simulink model "ALL_toghether"  (R2020b)
settings: Solver=ode1  StartTime=0.0  StopTime=50  FixedStep=0.001  RelTol=1e-3
values from neighbouring files (symbols this model uses):
  A = [0 -pi/16 0;pi/16 0 3*pi/16;0 0 0]    [feedbackControllerFinal.m]
  A_original1 = 1.2*A    [feedbackControllerFinal.m]
  A_original2 = 5*A    [feedbackControllerFinal.m]
  B = [1/2 1/2;0 0;1/0.15 -1/0.15]    [feedbackControllerFinal.m]
  C = [1 0 0;0 1 0]    [feedbackControllerFinal.m]
  F = -40    [feedbackControllerFinal.m]
  G_closeLoop = inv(C*inv(-(A-B*K1))*B)    [feedbackControllerFinal.m]
  K1 = place(A, B, [-30 -1+4.899*i -1-4.899*i])    [feedbackControllerFinal.m]
  K_f = K_bar(:,1:3)    [feedbackControllerFinal.m]
  Ka = K_bar(:,4:5)    [feedbackControllerFinal.m]
  L = L'    [feedbackControllerFinal.m]
  L_R = [1 -400]    [feedbackControllerFinal.m]
  Q1 = [1 0; 0 1; -0.5031 67.9061]    [feedbackControllerFinal.m]
  Q2 = [0 0 6.7909]'    [feedbackControllerFinal.m]
  T = lyap(-F, A, -L_R*C)    [feedbackControllerFinal.m]
settings Model: Creator=maral  LastModifiedBy=BALUCH
settings DebuggingCC: ArithmeticOperatorsInVariantConditions=warning
settings SFSimCC: CustomCodeUndefinedFunction=UseInterfaceOnly

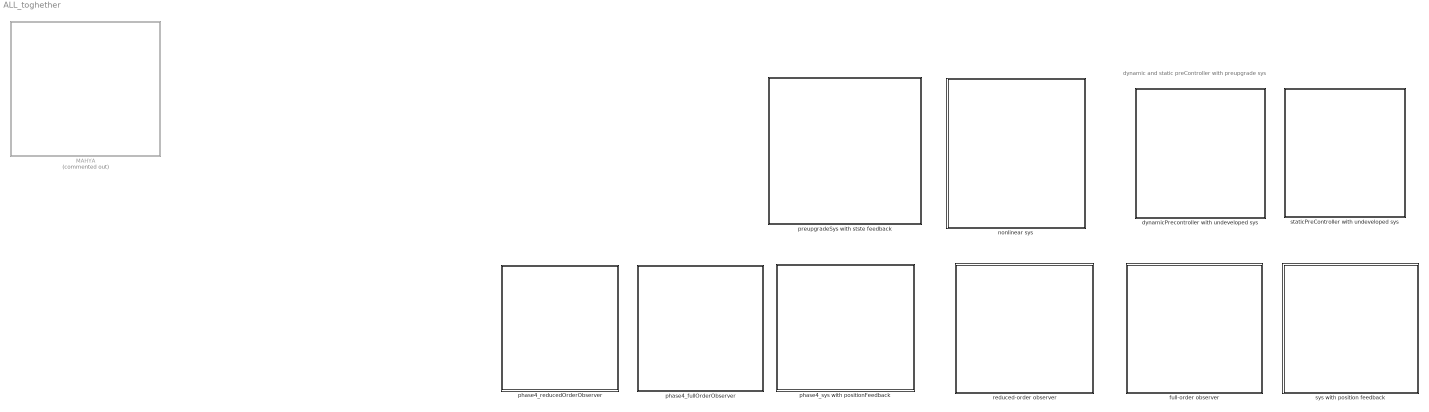
== system ALL_toghether ==
  note: dynamic and static preController with preupgrade sys
  "MAHYA " : Subsystem  Commented=on
  "dynamicPrecontroller with undeveloped sys " : Subsystem
  "full-order observer " : Subsystem
  "nonlinear sys " : Subsystem
  "phase4_fullOrderObserver " : Subsystem
  "phase4_reducedOrderObserver " : Subsystem
  "phase4_sys with positionFeedback " : Subsystem
  "preupgradeSys with stste feedback " : Subsystem
  reduced-order observer : Subsystem
  staticPreController with undeveloped sys : Subsystem
  sys with position feedback : Subsystem

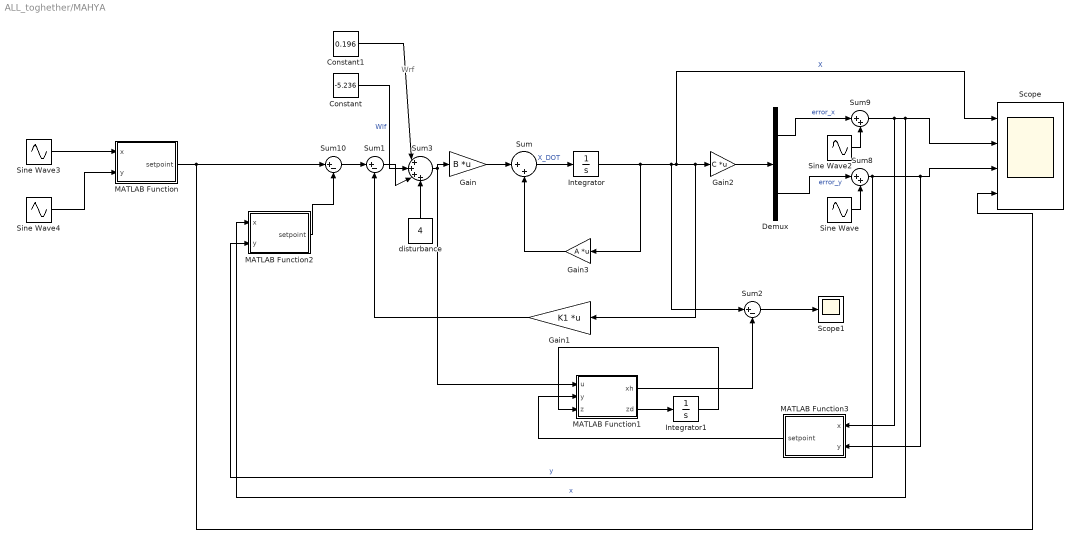
== system ALL_toghether/MAHYA  ==
  note: Wrf
  Constant : Constant  Value=-5.236
  Constant1 : Constant  Value=0.196
  Demux : Demux  Outputs=2
  Gain : Gain  Gain=B  Multiplication=Matrix(K*u)
  Gain1 : Gain  Gain=K1  Multiplication=Matrix(K*u)
  Gain2 : Gain  Gain=C  Multiplication=Matrix(K*u)
  Gain3 : Gain  Gain=A  Multiplication=Matrix(K*u)
  Integrator : Integrator
  Integrator1 : Integrator  InitialCondition=[0 0 0]
  MATLAB Function : MATLAB Function  TreatAsAtomicUnit=on
  MATLAB Function1 : MATLAB Function  TreatAsAtomicUnit=on
  MATLAB Function2 : MATLAB Function  TreatAsAtomicUnit=on
  MATLAB Function3 : MATLAB Function  TreatAsAtomicUnit=on
  Scope : Scope  NumInputPorts=4
  Scope1 : Scope
  Sine Wave : Sin  Amplitude=-3  Frequency=1/32  SampleTime=0
  Sine Wave2 : Sin  Amplitude=3  Frequency=1/32  Phase=pi/2  SampleTime=0
  Sine Wave3 : Sin  Amplitude=3  Frequency=1/30  Phase=pi/2  SampleTime=0
  Sine Wave4 : Sin  Amplitude=-3  Frequency=1/32  SampleTime=0
  Sum : Sum  Inputs=|++
  Sum1 : Sum  Inputs=|+-
  Sum10 : Sum  Inputs=|+-
  Sum2 : Sum  Inputs=|+-
  Sum3 : Sum  Inputs=|++++
  Sum8 : Sum  Inputs=|++
  Sum9 : Sum  Inputs=|++
  "disturbance " : Constant  Value=4
  wires:
  Demux/1 -> Sum9/1  "error_x"
  Sum9/1 -> MATLAB Function3/1(x), MATLAB Function2/1(x), Scope/2  "x"
  Gain3/1 -> Sum/2
  Sum8/1 -> MATLAB Function2/2(y), MATLAB Function3/2(y), Scope/3  "y"
  Gain2/1 -> Demux/1
  Sum10/1 -> Sum1/1
  MATLAB Function/1(setpoint) -> Scope/4, Sum10/1
  Integrator/1 -> Gain3/1, Sum2/1, Scope/1, Gain1/1, Gain2/1  "X"
  Gain/1 -> Sum/1
  Gain1/1 -> Sum1/2
  "disturbance "/1 -> Sum3/4
  Sum3/1 -> Gain/1, MATLAB Function1/1(u)
  Sine Wave/1 -> Sum8/2
  Sum/1 -> Integrator/1  "X_DOT"
  Sum1/1 -> Sum3/3
  Constant/1 -> Sum3/2  "Wlf"
  Sine Wave4/1 -> MATLAB Function/2(y)
  Sine Wave3/1 -> MATLAB Function/1(x)
  Sine Wave2/1 -> Sum9/2
  Constant1/1 -> Sum3/1
  MATLAB Function2/1(setpoint) -> Sum10/2
  Demux/2 -> Sum8/1  "error_y"
  MATLAB Function1/2(zd) -> Integrator1/1
  Integrator1/1 -> MATLAB Function1/3(z)
  MATLAB Function3/1(setpoint) -> MATLAB Function1/2(y)
  MATLAB Function1/1(xh) -> Sum2/2
  Sum2/1 -> Scope1/1

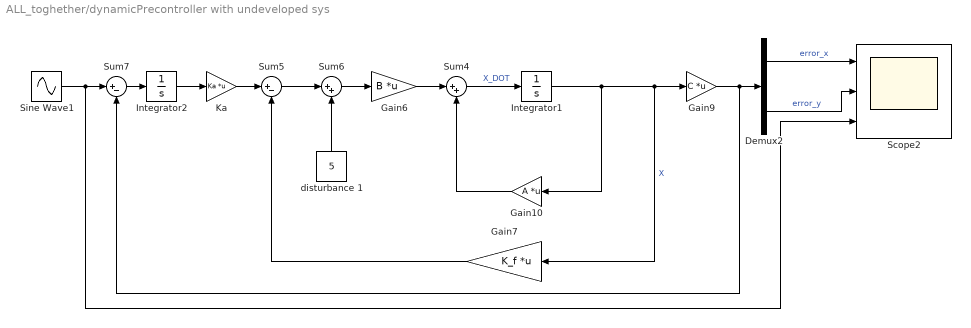
== system ALL_toghether/dynamicPrecontroller with undeveloped sys  ==
  Demux2 : Demux  Outputs=2
  Gain10 : Gain  Gain=A  Multiplication=Matrix(K*u)
  Gain6 : Gain  Gain=B  Multiplication=Matrix(K*u)
  Gain7 : Gain  Gain=K_f  Multiplication=Matrix(K*u)
  Gain9 : Gain  Gain=C  Multiplication=Matrix(K*u)
  Integrator1 : Integrator
  Integrator2 : Integrator
  "Ka " : Gain  Gain=Ka  Multiplication=Matrix(K*u)
  Scope2 : Scope  NumInputPorts=3
  Sine Wave1 : Sin  Amplitude=[1 1]  Bias=[0 0]  Frequency=[1 1]  SampleTime=0
  Sum4 : Sum  Inputs=|++
  Sum5 : Sum  Inputs=|+-
  Sum6 : Sum  Inputs=|++
  Sum7 : Sum  Inputs=|+-
  disturbance 1 : Constant  Value=5
  wires:
  Sum5/1 -> Sum6/1
  Integrator2/1 -> "Ka "/1
  Sum7/1 -> Integrator2/1
  disturbance 1/1 -> Sum6/2
  Integrator1/1 -> Gain10/1, Gain7/1, Gain9/1  "X"
  Gain7/1 -> Sum5/2
  Gain6/1 -> Sum4/1
  Gain10/1 -> Sum4/2
  Sine Wave1/1 -> Scope2/3, Sum7/1
  Demux2/2 -> Scope2/2  "error_y"
  "Ka "/1 -> Sum5/1
  Sum6/1 -> Gain6/1
  Demux2/1 -> Scope2/1  "error_x"
  Gain9/1 -> Sum7/2, Demux2/1
  Sum4/1 -> Integrator1/1  "X_DOT"

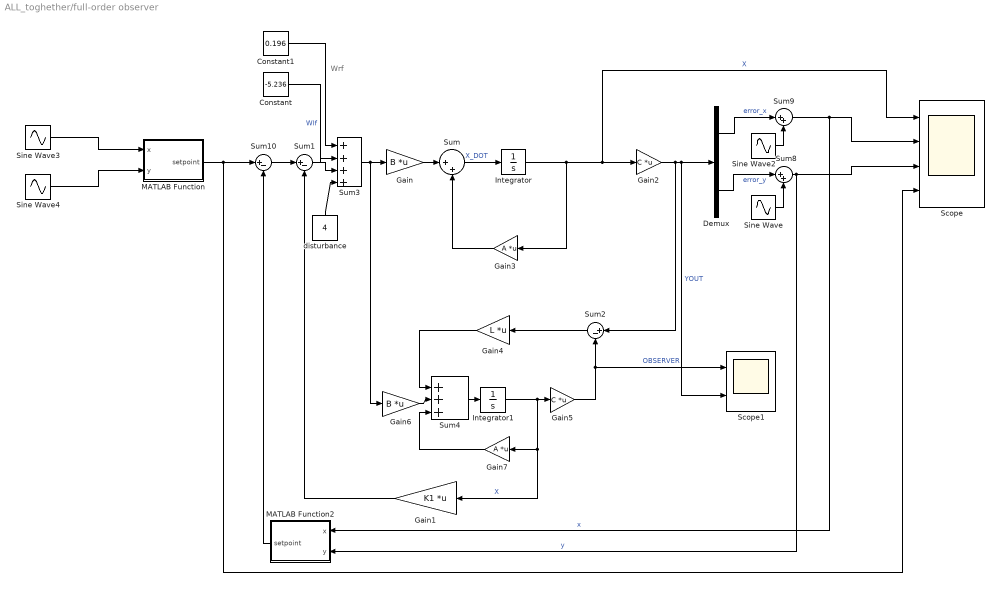
== system ALL_toghether/full-order observer  ==
  note: Wrf
  Constant : Constant  Value=-5.236
  Constant1 : Constant  Value=0.196
  Demux : Demux  Outputs=2
  Gain : Gain  Gain=B  Multiplication=Matrix(K*u)
  Gain1 : Gain  Gain=K1  Multiplication=Matrix(K*u)
  Gain2 : Gain  Gain=C  Multiplication=Matrix(K*u)
  Gain3 : Gain  Gain=A  Multiplication=Matrix(K*u)
  Gain4 : Gain  Gain=L  Multiplication=Matrix(K*u)
  Gain5 : Gain  Gain=C  Multiplication=Matrix(K*u)
  Gain6 : Gain  Gain=B  Multiplication=Matrix(K*u)
  Gain7 : Gain  Gain=A  Multiplication=Matrix(K*u)
  Integrator : Integrator  InitialCondition=[0.1 0.1 0]'
  Integrator1 : Integrator  InitialCondition=[0.4 0.4 0.5]'
  MATLAB Function : MATLAB Function  TreatAsAtomicUnit=on
  MATLAB Function2 : MATLAB Function  TreatAsAtomicUnit=on
  Scope : Scope  NumInputPorts=4
  Scope1 : Scope  NumInputPorts=2
  Sine Wave : Sin  Amplitude=-3  Frequency=pi/16  SampleTime=0
  Sine Wave2 : Sin  Amplitude=3  Frequency=pi/16  Phase=pi/2  SampleTime=0
  Sine Wave3 : Sin  Amplitude=3  Frequency=pi/16  Phase=pi/2  SampleTime=0
  Sine Wave4 : Sin  Amplitude=-3  Frequency=pi/16  SampleTime=0
  Sum : Sum  Inputs=|++
  Sum1 : Sum  Inputs=|+-
  Sum10 : Sum  Inputs=|+-
  Sum2 : Sum  Inputs=|+-
  Sum3 : Sum  Inputs=|++++
  Sum4 : Sum  Inputs=|+++
  Sum8 : Sum  Inputs=|++
  Sum9 : Sum  Inputs=|++
  "disturbance " : Constant  Value=4
  wires:
  Sum8/1 -> MATLAB Function2/2(y), Scope/3  "y"
  Constant/1 -> Sum3/2  "Wlf"
  Sum10/1 -> Sum1/1
  Sine Wave/1 -> Sum8/2
  Integrator/1 -> Gain3/1, Scope/1, Gain2/1  "X"
  Gain1/1 -> Sum1/2
  Demux/1 -> Sum9/1  "error_x"
  "disturbance "/1 -> Sum3/4
  Sum9/1 -> MATLAB Function2/1(x), Scope/2  "x"
  MATLAB Function/1(setpoint) -> Scope/4, Sum10/1
  Constant1/1 -> Sum3/1
  Sine Wave2/1 -> Sum9/2
  Sum3/1 -> Gain6/1, Gain/1
  Gain3/1 -> Sum/2
  Gain2/1 -> Sum2/1, Scope1/2, Demux/1  "YOUT"
  Sum1/1 -> Sum3/3
  Sine Wave3/1 -> MATLAB Function/1(x)
  Gain/1 -> Sum/1
  MATLAB Function2/1(setpoint) -> Sum10/2
  Demux/2 -> Sum8/1  "error_y"
  Sine Wave4/1 -> MATLAB Function/2(y)
  Sum/1 -> Integrator/1  "X_DOT"
  Gain5/1 -> Sum2/2, Scope1/1  "OBSERVER"
  Integrator1/1 -> Gain7/1, Gain1/1, Gain5/1  "X"
  Sum4/1 -> Integrator1/1
  Gain6/1 -> Sum4/2
  Gain4/1 -> Sum4/1
  Gain7/1 -> Sum4/3
  Sum2/1 -> Gain4/1

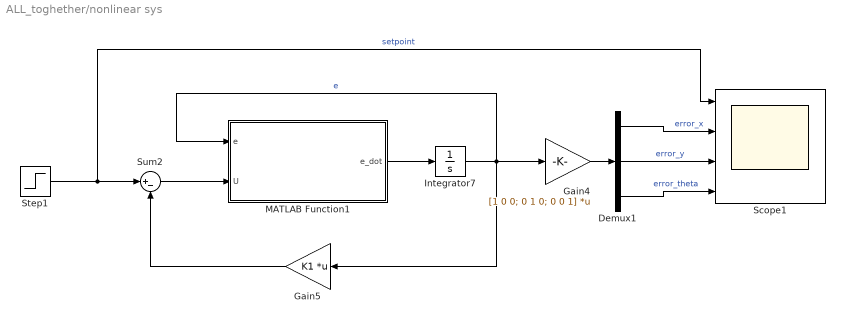
== system ALL_toghether/nonlinear sys  ==
  Demux1 : Demux  Outputs=3
  Gain4 : Gain  Gain=[1 0 0; 0 1 0; 0 0 1]  Multiplication=Matrix(K*u)
  Gain5 : Gain  Gain=K1  Multiplication=Matrix(K*u)
  Integrator7 : Integrator  InitialCondition=[0.45; -0.3; -0.3]
  MATLAB Function1 : MATLAB Function  TreatAsAtomicUnit=on
  Scope1 : Scope  NumInputPorts=4
  Step1 : Step  Time=[0;0]  Before=[0;0]  After=[0.1;0.2]  SampleTime=0
  Sum2 : Sum  Inputs=|+-
  wires:
  Sum2/1 -> MATLAB Function1/2(U)
  Gain5/1 -> Sum2/2
  Integrator7/1 -> MATLAB Function1/1(e), Gain4/1, Gain5/1  "e"
  MATLAB Function1/1(e_dot) -> Integrator7/1
  Gain4/1 -> Demux1/1
  Demux1/1 -> Scope1/2  "error_x"
  Step1/1 -> Sum2/1, Scope1/1  "setpoint"
  Demux1/2 -> Scope1/3  "error_y"
  Demux1/3 -> Scope1/4  "error_theta"

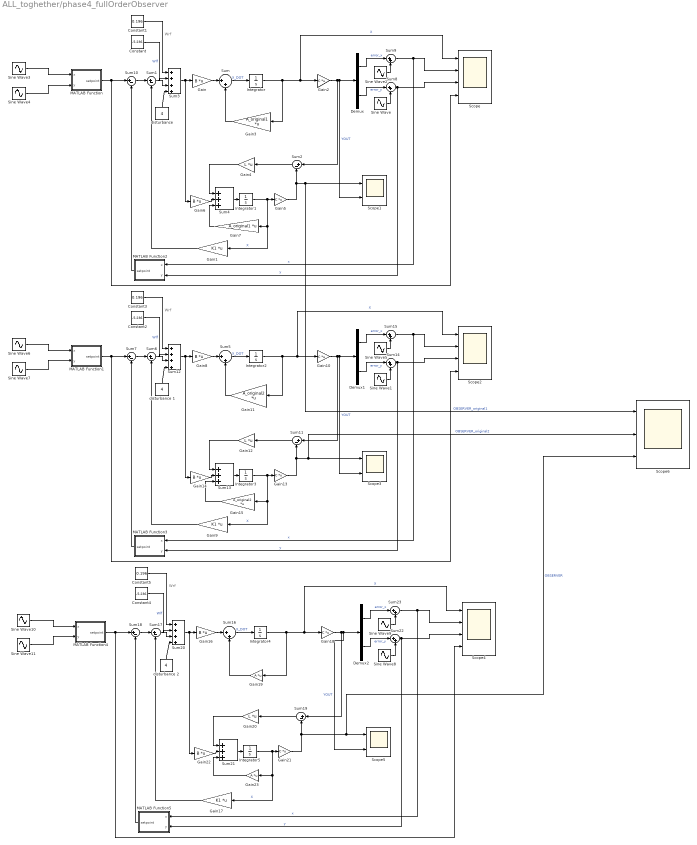
== system ALL_toghether/phase4_fullOrderObserver  ==
  note: Wrf
  note: Wrf
  note: Wrf
  Constant : Constant  Value=-5.236
  Constant1 : Constant  Value=0.196
  Constant2 : Constant  Value=-5.236
  Constant3 : Constant  Value=0.196
  Constant4 : Constant  Value=-5.236
  Constant5 : Constant  Value=0.196
  Demux : Demux  Outputs=2
  Demux1 : Demux  Outputs=2
  Demux2 : Demux  Outputs=2
  Gain{,6,8,14,16,22} (6 alike) : Gain  Gain=B  Multiplication=Matrix(K*u)
  Gain1 : Gain  Gain=K1  Multiplication=Matrix(K*u)
  Gain{2,5,10,13,18,21} (6 alike) : Gain  Gain=C  Multiplication=Matrix(K*u)
  Gain11 : Gain  Gain=A_original2  Multiplication=Matrix(K*u)
  Gain12 : Gain  Gain=L  Multiplication=Matrix(K*u)
  Gain15 : Gain  Gain=A_original2  Multiplication=Matrix(K*u)
  Gain17 : Gain  Gain=K1  Multiplication=Matrix(K*u)
  Gain19 : Gain  Gain=A  Multiplication=Matrix(K*u)
  Gain20 : Gain  Gain=L  Multiplication=Matrix(K*u)
  Gain23 : Gain  Gain=A  Multiplication=Matrix(K*u)
  Gain3 : Gain  Gain=A_original1  Multiplication=Matrix(K*u)
  Gain4 : Gain  Gain=L  Multiplication=Matrix(K*u)
  Gain7 : Gain  Gain=A_original1  Multiplication=Matrix(K*u)
  Gain9 : Gain  Gain=K1  Multiplication=Matrix(K*u)
  Integrator : Integrator  InitialCondition=[0.1 0.1 0]'
  Integrator1 : Integrator  InitialCondition=[0.4 0.4 0.5]'
  Integrator2 : Integrator  InitialCondition=[0.1 0.1 0]'
  Integrator3 : Integrator  InitialCondition=[0.4 0.4 0.5]'
  Integrator4 : Integrator  InitialCondition=[0.1 0.1 0]'
  Integrator5 : Integrator  InitialCondition=[0.4 0.4 0.5]'
  MATLAB Function : MATLAB Function  TreatAsAtomicUnit=on
  MATLAB Function1 : MATLAB Function  TreatAsAtomicUnit=on
  MATLAB Function2 : MATLAB Function  TreatAsAtomicUnit=on
  MATLAB Function3 : MATLAB Function  TreatAsAtomicUnit=on
  MATLAB Function4 : MATLAB Function  TreatAsAtomicUnit=on
  MATLAB Function5 : MATLAB Function  TreatAsAtomicUnit=on
  Scope : Scope  NumInputPorts=4
  Scope1 : Scope  NumInputPorts=2
  Scope2 : Scope  NumInputPorts=4
  Scope3 : Scope  NumInputPorts=2
  Scope4 : Scope  NumInputPorts=4
  Scope5 : Scope  NumInputPorts=2
  Scope6 : Scope  NumInputPorts=3
  Sine Wave{,1,4,7..8,11} (6 alike) : Sin  Amplitude=-3  Frequency=pi/16  SampleTime=0
  Sine Wave{2..3,5..6,9..10} (6 alike) : Sin  Amplitude=3  Frequency=pi/16  Phase=pi/2  SampleTime=0
  Sum{,5,8..9,14..16,22..23} (9 alike) : Sum  Inputs=|++
  Sum{1..2,6..7,10..11,17..19} (9 alike) : Sum  Inputs=|+-
  Sum12 : Sum  Inputs=|++++
  Sum13 : Sum  Inputs=|+++
  Sum20 : Sum  Inputs=|++++
  Sum21 : Sum  Inputs=|+++
  Sum3 : Sum  Inputs=|++++
  Sum4 : Sum  Inputs=|+++
  "disturbance " : Constant  Value=4
  disturbance 1 : Constant  Value=4
  disturbance 2 : Constant  Value=4
  wires:
  MATLAB Function2/1(setpoint) -> Sum10/2
  Gain7/1 -> Sum4/3
  Gain4/1 -> Sum4/1
  Sine Wave2/1 -> Sum9/2
  Gain2/1 -> Sum2/1, Scope1/2, Demux/1  "YOUT"
  Sum8/1 -> MATLAB Function2/2(y), Scope/3  "y"
  Gain5/1 -> Sum2/2, Scope6/1, Scope1/1  "OBSERVER_original1"
  "disturbance "/1 -> Sum3/4
  Sum9/1 -> MATLAB Function2/1(x), Scope/2  "x"
  Gain/1 -> Sum/1
  Gain6/1 -> Sum4/2
  Sine Wave4/1 -> MATLAB Function/2(y)
  Sum2/1 -> Gain4/1
  Sum3/1 -> Gain6/1, Gain/1
  Sum/1 -> Integrator/1  "X_DOT"
  Sum10/1 -> Sum1/1
  Gain3/1 -> Sum/2
  Constant/1 -> Sum3/2  "Wlf"
  Sum4/1 -> Integrator1/1
  Sine Wave3/1 -> MATLAB Function/1(x)
  MATLAB Function/1(setpoint) -> Scope/4, Sum10/1
  Demux/1 -> Sum9/1  "error_x"
  Integrator1/1 -> Gain7/1, Gain1/1, Gain5/1  "X"
  Sum1/1 -> Sum3/3
  Integrator/1 -> Gain3/1, Scope/1, Gain2/1  "X"
  Demux/2 -> Sum8/1  "error_y"
  Gain1/1 -> Sum1/2
  Sine Wave/1 -> Sum8/2
  Constant1/1 -> Sum3/1
  Sum11/1 -> Gain12/1
  Sine Wave7/1 -> MATLAB Function1/2(y)
  Sum5/1 -> Integrator2/1  "X_DOT"
  Sum7/1 -> Sum6/1
  Sum15/1 -> MATLAB Function3/1(x), Scope2/2  "x"
  disturbance 1/1 -> Sum12/4
  Gain13/1 -> Sum11/2, Scope6/2, Scope3/1  "OBSERVER_original2"
  Sum14/1 -> MATLAB Function3/2(y), Scope2/3  "y"
  Gain12/1 -> Sum13/1
  Sine Wave5/1 -> Sum15/2
  Constant3/1 -> Sum12/1
  Gain15/1 -> Sum13/3
  MATLAB Function3/1(setpoint) -> Sum7/2
  Gain10/1 -> Sum11/1, Scope3/2, Demux1/1  "YOUT"
  Gain9/1 -> Sum6/2
  Integrator2/1 -> Gain11/1, Scope2/1, Gain10/1  "X"
  Demux1/2 -> Sum14/1  "error_y"
  Sum13/1 -> Integrator3/1
  Sine Wave1/1 -> Sum14/2
  Integrator3/1 -> Gain15/1, Gain9/1, Gain13/1  "X"
  Sum12/1 -> Gain14/1, Gain8/1
  Sum6/1 -> Sum12/3
  Sine Wave6/1 -> MATLAB Function1/1(x)
  MATLAB Function1/1(setpoint) -> Scope2/4, Sum7/1
  Gain8/1 -> Sum5/1
  Gain14/1 -> Sum13/2
  Constant2/1 -> Sum12/2  "Wlf"
  Gain11/1 -> Sum5/2
  Demux1/1 -> Sum15/1  "error_x"
  Sum19/1 -> Gain20/1
  Sine Wave11/1 -> MATLAB Function4/2(y)
  Sum16/1 -> Integrator4/1  "X_DOT"
  Sum18/1 -> Sum17/1
  Sum23/1 -> MATLAB Function5/1(x), Scope4/2  "x"
  disturbance 2/1 -> Sum20/4
  Gain21/1 -> Sum19/2, Scope6/3, Scope5/1  "OBSERVER"
  Sum22/1 -> MATLAB Function5/2(y), Scope4/3  "y"
  Gain20/1 -> Sum21/1
  Sine Wave9/1 -> Sum23/2
  Constant5/1 -> Sum20/1
  Gain23/1 -> Sum21/3
  MATLAB Function5/1(setpoint) -> Sum18/2
  Gain18/1 -> Sum19/1, Scope5/2, Demux2/1  "YOUT"
  Gain17/1 -> Sum17/2
  Integrator4/1 -> Gain19/1, Scope4/1, Gain18/1  "X"
  Demux2/2 -> Sum22/1  "error_y"
  Sum21/1 -> Integrator5/1
  Sine Wave8/1 -> Sum22/2
  Integrator5/1 -> Gain23/1, Gain17/1, Gain21/1  "X"
  Sum20/1 -> Gain22/1, Gain16/1
  Sum17/1 -> Sum20/3
  Sine Wave10/1 -> MATLAB Function4/1(x)
  MATLAB Function4/1(setpoint) -> Scope4/4, Sum18/1
  Gain16/1 -> Sum16/1
  Gain22/1 -> Sum21/2
  Constant4/1 -> Sum20/2  "Wlf"
  Gain19/1 -> Sum16/2
  Demux2/1 -> Sum23/1  "error_x"

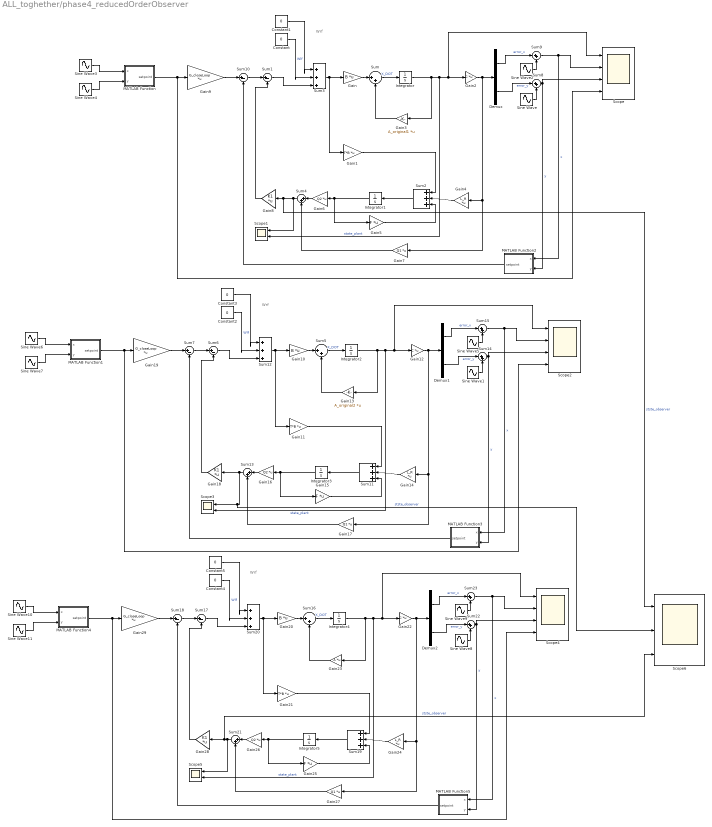
== system ALL_toghether/phase4_reducedOrderObserver  ==
  note: Wrf
  note: Wrf
  note: Wrf
  Constant{,1..5} (6 alike) : Constant  Value=0
  Demux : Demux  Outputs=2
  Demux1 : Demux  Outputs=2
  Demux2 : Demux  Outputs=2
  Gain : Gain  Gain=B  Multiplication=Matrix(K*u)
  Gain1 : Gain  Gain=T*B  Multiplication=Matrix(K*u)
  Gain10 : Gain  Gain=B  Multiplication=Matrix(K*u)
  Gain11 : Gain  Gain=T*B  Multiplication=Matrix(K*u)
  Gain12 : Gain  Gain=C  Multiplication=Matrix(K*u)
  Gain13 : Gain  Gain=A_original2  Multiplication=Matrix(K*u)
  Gain14 : Gain  Gain=L_R  Multiplication=Matrix(K*u)
  Gain15 : Gain  Gain=F  Multiplication=Matrix(K*u)
  Gain16 : Gain  Gain=Q2  Multiplication=Matrix(K*u)
  Gain17 : Gain  Gain=Q1  Multiplication=Matrix(K*u)
  Gain18 : Gain  Gain=K1  Multiplication=Matrix(K*u)
  Gain19 : Gain  Gain=G_closeLoop  Multiplication=Matrix(K*u)
  Gain2 : Gain  Gain=C  Multiplication=Matrix(K*u)
  Gain20 : Gain  Gain=B  Multiplication=Matrix(K*u)
  Gain21 : Gain  Gain=T*B  Multiplication=Matrix(K*u)
  Gain22 : Gain  Gain=C  Multiplication=Matrix(K*u)
  Gain23 : Gain  Gain=A  Multiplication=Matrix(K*u)
  Gain24 : Gain  Gain=L_R  Multiplication=Matrix(K*u)
  Gain25 : Gain  Gain=F  Multiplication=Matrix(K*u)
  Gain26 : Gain  Gain=Q2  Multiplication=Matrix(K*u)
  Gain27 : Gain  Gain=Q1  Multiplication=Matrix(K*u)
  Gain28 : Gain  Gain=K1  Multiplication=Matrix(K*u)
  Gain29 : Gain  Gain=G_closeLoop  Multiplication=Matrix(K*u)
  Gain3 : Gain  Gain=A_original1  Multiplication=Matrix(K*u)
  Gain4 : Gain  Gain=L_R  Multiplication=Matrix(K*u)
  Gain5 : Gain  Gain=F  Multiplication=Matrix(K*u)
  Gain6 : Gain  Gain=Q2  Multiplication=Matrix(K*u)
  Gain7 : Gain  Gain=Q1  Multiplication=Matrix(K*u)
  Gain8 : Gain  Gain=K1  Multiplication=Matrix(K*u)
  Gain9 : Gain  Gain=G_closeLoop  Multiplication=Matrix(K*u)
  Integrator : Integrator  InitialCondition=[0.1 0.1 0]'
  Integrator1 : Integrator  InitialCondition=0.05
  Integrator2 : Integrator  InitialCondition=[0.1 0.1 0]'
  Integrator3 : Integrator
  Integrator4 : Integrator  InitialCondition=[0.1 0.1 0]'
  Integrator5 : Integrator
  MATLAB Function : MATLAB Function  TreatAsAtomicUnit=on
  MATLAB Function1 : MATLAB Function  TreatAsAtomicUnit=on
  MATLAB Function2 : MATLAB Function  TreatAsAtomicUnit=on
  MATLAB Function3 : MATLAB Function  TreatAsAtomicUnit=on
  MATLAB Function4 : MATLAB Function  TreatAsAtomicUnit=on
  MATLAB Function5 : MATLAB Function  TreatAsAtomicUnit=on
  Scope : Scope  NumInputPorts=4
  Scope1 : Scope  NumInputPorts=2
  Scope2 : Scope  NumInputPorts=4
  Scope3 : Scope  NumInputPorts=2
  Scope4 : Scope  NumInputPorts=4
  Scope5 : Scope  NumInputPorts=2
  Scope6 : Scope  NumInputPorts=3
  Sine Wave{,1,4,7..8,11} (6 alike) : Sin  Amplitude=-3  Frequency=pi/16  SampleTime=0
  Sine Wave{2..3,5..6,9..10} (6 alike) : Sin  Amplitude=3  Frequency=pi/16  Phase=pi/2  SampleTime=0
  Sum{,4..5,8..9,13..16,21..23} (12 alike) : Sum  Inputs=|++
  Sum{1,6..7,10,17..18} (6 alike) : Sum  Inputs=|+-
  Sum{2..3,11..12,19..20} (6 alike) : Sum  Inputs=|+++
  wires:
  Sine Wave3/1 -> MATLAB Function/1(x)
  Integrator/1 -> Gain3/1, Scope1/2, Scope/1, Gain2/1  "state_plant"
  Gain5/1 -> Sum2/3
  MATLAB Function/1(setpoint) -> Scope/4, Gain9/1
  Sine Wave4/1 -> MATLAB Function/2(y)
  Sum3/1 -> Gain1/1, Gain/1
  Sum4/1 -> Scope1/1, Scope6/1, Gain8/1  "stste_observer"
  Gain9/1 -> Sum10/1
  Constant1/1 -> Sum3/1
  Gain/1 -> Sum/1
  Sum8/1 -> MATLAB Function2/2(y), Scope/3  "y"
  Sine Wave/1 -> Sum8/2
  Constant/1 -> Sum3/2  "Wlf"
  Integrator1/1 -> Gain5/1, Gain6/1
  Gain7/1 -> Sum4/2
  Gain1/1 -> Sum2/1
  Gain3/1 -> Sum/2
  Sine Wave2/1 -> Sum9/2
  Sum2/1 -> Integrator1/1
  Gain4/1 -> Sum2/2
  Demux/2 -> Sum8/1  "error_y"
  Gain2/1 -> Gain7/1, Gain4/1, Demux/1
  Demux/1 -> Sum9/1  "error_x"
  Gain6/1 -> Sum4/1
  Gain8/1 -> Sum1/2
  Sum9/1 -> MATLAB Function2/1(x), Scope/2  "x"
  Sum1/1 -> Sum3/3
  MATLAB Function2/1(setpoint) -> Sum10/2
  Sum/1 -> Integrator/1  "X_DOT"
  Sum10/1 -> Sum1/1
  Sum7/1 -> Sum6/1
  Sum5/1 -> Integrator2/1  "X_DOT"
  Sum15/1 -> MATLAB Function3/1(x), Scope2/2  "x"
  MATLAB Function3/1(setpoint) -> Sum7/2
  Sum6/1 -> Sum12/3
  Gain12/1 -> Gain17/1, Gain14/1, Demux1/1
  Demux1/1 -> Sum15/1  "error_x"
  Sum11/1 -> Integrator3/1
  Gain16/1 -> Sum13/1
  Demux1/2 -> Sum14/1  "error_y"
  Gain14/1 -> Sum11/2
  Integrator3/1 -> Gain15/1, Gain16/1
  Gain11/1 -> Sum11/1
  Gain13/1 -> Sum5/2
  Constant2/1 -> Sum12/2  "Wlf"
  Sum14/1 -> MATLAB Function3/2(y), Scope2/3  "y"
  Sine Wave6/1 -> MATLAB Function1/1(x)
  Sine Wave5/1 -> Sum15/2
  Gain15/1 -> Sum11/3
  Sine Wave7/1 -> MATLAB Function1/2(y)
  Integrator2/1 -> Gain13/1, Scope3/2, Scope2/1, Gain12/1  "state_plant"
  Gain18/1 -> Sum6/2
  Sum12/1 -> Gain11/1, Gain10/1
  MATLAB Function1/1(setpoint) -> Scope2/4, Gain19/1
  Gain19/1 -> Sum7/1
  Constant3/1 -> Sum12/1
  Sum13/1 -> Scope3/1, Scope6/2, Gain18/1  "stste_observer"
  Gain17/1 -> Sum13/2
  Gain10/1 -> Sum5/1
  Sine Wave1/1 -> Sum14/2
  Sum18/1 -> Sum17/1
  Sum16/1 -> Integrator4/1  "X_DOT"
  Sum23/1 -> MATLAB Function5/1(x), Scope4/2  "x"
  MATLAB Function5/1(setpoint) -> Sum18/2
  Sum17/1 -> Sum20/3
  Gain22/1 -> Gain27/1, Gain24/1, Demux2/1
  Demux2/1 -> Sum23/1  "error_x"
  Sum19/1 -> Integrator5/1
  Gain26/1 -> Sum21/1
  Demux2/2 -> Sum22/1  "error_y"
  Gain24/1 -> Sum19/2
  Integrator5/1 -> Gain25/1, Gain26/1
  Gain21/1 -> Sum19/1
  Gain23/1 -> Sum16/2
  Constant4/1 -> Sum20/2  "Wlf"
  Sum22/1 -> MATLAB Function5/2(y), Scope4/3  "y"
  Sine Wave10/1 -> MATLAB Function4/1(x)
  Sine Wave9/1 -> Sum23/2
  Gain25/1 -> Sum19/3
  Sine Wave11/1 -> MATLAB Function4/2(y)
  Integrator4/1 -> Gain23/1, Scope5/2, Scope4/1, Gain22/1  "state_plant"
  Gain28/1 -> Sum17/2
  Sum20/1 -> Gain21/1, Gain20/1
  MATLAB Function4/1(setpoint) -> Scope4/4, Gain29/1
  Gain29/1 -> Sum18/1
  Constant5/1 -> Sum20/1
  Sum21/1 -> Scope5/1, Scope6/3, Gain28/1  "stste_observer"
  Gain27/1 -> Sum21/2
  Gain20/1 -> Sum16/1
  Sine Wave8/1 -> Sum22/2

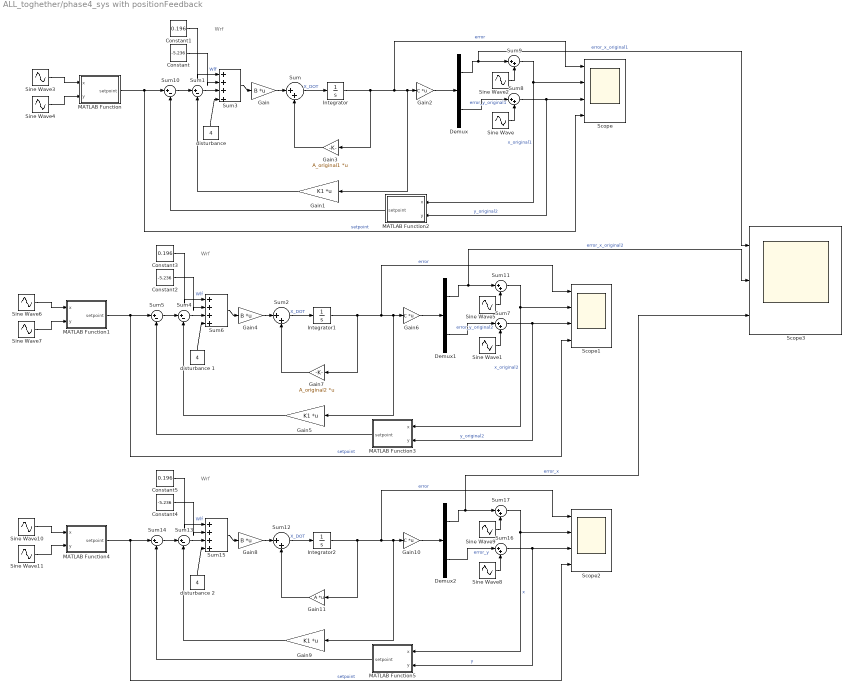
== system ALL_toghether/phase4_sys with positionFeedback  ==
  note: Wrf
  note: Wrf
  note: Wrf
  Constant : Constant  Value=-5.236
  Constant1 : Constant  Value=0.196
  Constant2 : Constant  Value=-5.236
  Constant3 : Constant  Value=0.196
  Constant4 : Constant  Value=-5.236
  Constant5 : Constant  Value=0.196
  Demux : Demux  Outputs=2
  Demux1 : Demux  Outputs=2
  Demux2 : Demux  Outputs=2
  Gain : Gain  Gain=B  Multiplication=Matrix(K*u)
  Gain1 : Gain  Gain=K1  Multiplication=Matrix(K*u)
  Gain10 : Gain  Gain=C  Multiplication=Matrix(K*u)
  Gain11 : Gain  Gain=A  Multiplication=Matrix(K*u)
  Gain2 : Gain  Gain=C  Multiplication=Matrix(K*u)
  Gain3 : Gain  Gain=A_original1  Multiplication=Matrix(K*u)
  Gain4 : Gain  Gain=B  Multiplication=Matrix(K*u)
  Gain5 : Gain  Gain=K1  Multiplication=Matrix(K*u)
  Gain6 : Gain  Gain=C  Multiplication=Matrix(K*u)
  Gain7 : Gain  Gain=A_original2  Multiplication=Matrix(K*u)
  Gain8 : Gain  Gain=B  Multiplication=Matrix(K*u)
  Gain9 : Gain  Gain=K1  Multiplication=Matrix(K*u)
  Integrator : Integrator  InitialCondition=[0.1; 0.1; 0.1]
  Integrator1 : Integrator  InitialCondition=[0.1; 0.1; 0.1]
  Integrator2 : Integrator  InitialCondition=[0.1; 0.1; 0.1]
  MATLAB Function : MATLAB Function  TreatAsAtomicUnit=on
  MATLAB Function1 : MATLAB Function  TreatAsAtomicUnit=on
  MATLAB Function2 : MATLAB Function  TreatAsAtomicUnit=on
  MATLAB Function3 : MATLAB Function  TreatAsAtomicUnit=on
  MATLAB Function4 : MATLAB Function  TreatAsAtomicUnit=on
  MATLAB Function5 : MATLAB Function  TreatAsAtomicUnit=on
  Scope : Scope  NumInputPorts=4
  Scope1 : Scope  NumInputPorts=4
  Scope2 : Scope  NumInputPorts=4
  Scope3 : Scope  NumInputPorts=3
  Sine Wave{,1,4,7..8,11} (6 alike) : Sin  Amplitude=-3  Frequency=pi/16  SampleTime=0
  Sine Wave{2..3,5..6,9..10} (6 alike) : Sin  Amplitude=3  Frequency=pi/16  Phase=pi/2  SampleTime=0
  Sum{,2,7..9,11..12,16..17} (9 alike) : Sum  Inputs=|++
  Sum{1,4..5,10,13..14} (6 alike) : Sum  Inputs=|+-
  Sum15 : Sum  Inputs=|++++
  Sum3 : Sum  Inputs=|++++
  Sum6 : Sum  Inputs=|++++
  "disturbance " : Constant  Value=4
  disturbance 1 : Constant  Value=4
  disturbance 2 : Constant  Value=4
  wires:
  Demux/2 -> Sum8/1  "error_y_original1"
  Sine Wave/1 -> Sum8/2
  Sine Wave2/1 -> Sum9/2
  Gain2/1 -> Demux/1
  MATLAB Function/1(setpoint) -> Sum10/1, Scope/4  "setpoint"
  Sine Wave4/1 -> MATLAB Function/2(y)
  "disturbance "/1 -> Sum3/4
  MATLAB Function2/1(setpoint) -> Sum10/2
  Sum/1 -> Integrator/1  "X_DOT"
  Gain3/1 -> Sum/2
  Sine Wave3/1 -> MATLAB Function/1(x)
  Sum8/1 -> Scope/3, MATLAB Function2/2(y)  "y_original2"
  Constant1/1 -> Sum3/1
  Sum9/1 -> Scope/2, MATLAB Function2/1(x)  "x_original1"
  Sum10/1 -> Sum1/1
  Demux/1 -> Scope3/1, Sum9/1  "error_x_original1"
  Gain1/1 -> Sum1/2
  Sum1/1 -> Sum3/3
  Constant/1 -> Sum3/2  "Wlf"
  Gain/1 -> Sum/1
  Integrator/1 -> Gain2/1, Gain1/1, Scope/1, Gain3/1  "error"
  Sum3/1 -> Gain/1
  Integrator1/1 -> Gain6/1, Gain5/1, Scope1/1, Gain7/1  "error"
  Sum6/1 -> Gain4/1
  Sum2/1 -> Integrator1/1  "X_DOT"
  Demux1/1 -> Scope3/2, Sum11/1  "error_x_original2"
  Sum11/1 -> Scope1/2, MATLAB Function3/1(x)  "x_original2"
  Sum5/1 -> Sum4/1
  Constant3/1 -> Sum6/1
  Gain7/1 -> Sum2/2
  Sum4/1 -> Sum6/3
  Gain5/1 -> Sum4/2
  Demux1/2 -> Sum7/1  "error_y_original2"
  Sine Wave1/1 -> Sum7/2
  Sum7/1 -> Scope1/3, MATLAB Function3/2(y)  "y_original2"
  MATLAB Function3/1(setpoint) -> Sum5/2
  MATLAB Function1/1(setpoint) -> Sum5/1, Scope1/4  "setpoint"
  Gain6/1 -> Demux1/1
  Sine Wave5/1 -> Sum11/2
  Sine Wave7/1 -> MATLAB Function1/2(y)
  Gain4/1 -> Sum2/1
  Constant2/1 -> Sum6/2  "Wlf"
  Sine Wave6/1 -> MATLAB Function1/1(x)
  disturbance 1/1 -> Sum6/4
  Integrator2/1 -> Gain10/1, Gain9/1, Scope2/1, Gain11/1  "error"
  Sum15/1 -> Gain8/1
  Sum12/1 -> Integrator2/1  "X_DOT"
  Demux2/1 -> Scope3/3, Sum17/1  "error_x"
  Sum17/1 -> Scope2/2, MATLAB Function5/1(x)  "x"
  Sum14/1 -> Sum13/1
  Constant5/1 -> Sum15/1
  Gain11/1 -> Sum12/2
  Sum13/1 -> Sum15/3
  Gain9/1 -> Sum13/2
  Demux2/2 -> Sum16/1  "error_y"
  Sine Wave8/1 -> Sum16/2
  Sum16/1 -> Scope2/3, MATLAB Function5/2(y)  "y"
  MATLAB Function5/1(setpoint) -> Sum14/2
  MATLAB Function4/1(setpoint) -> Sum14/1, Scope2/4  "setpoint"
  Gain10/1 -> Demux2/1
  Sine Wave9/1 -> Sum17/2
  Sine Wave11/1 -> MATLAB Function4/2(y)
  Gain8/1 -> Sum12/1
  Constant4/1 -> Sum15/2  "Wlf"
  Sine Wave10/1 -> MATLAB Function4/1(x)
  disturbance 2/1 -> Sum15/4

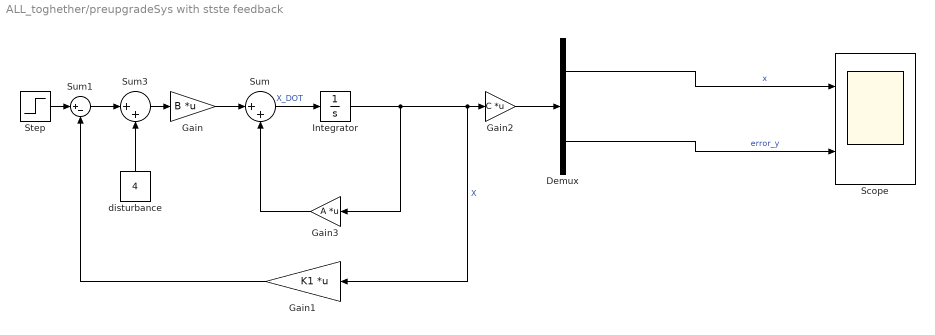
== system ALL_toghether/preupgradeSys with stste feedback  ==
  Demux : Demux  Outputs=2
  Gain : Gain  Gain=B  Multiplication=Matrix(K*u)
  Gain1 : Gain  Gain=K1  Multiplication=Matrix(K*u)
  Gain2 : Gain  Gain=C  Multiplication=Matrix(K*u)
  Gain3 : Gain  Gain=A  Multiplication=Matrix(K*u)
  Integrator : Integrator
  Scope : Scope  NumInputPorts=2
  Step : Step  SampleTime=0
  Sum : Sum  Inputs=|++
  Sum1 : Sum  Inputs=|+-
  Sum3 : Sum  Inputs=|++
  "disturbance " : Constant  Value=4
  wires:
  Gain3/1 -> Sum/2
  Sum/1 -> Integrator/1  "X_DOT"
  Sum3/1 -> Gain/1
  Gain/1 -> Sum/1
  Gain1/1 -> Sum1/2
  "disturbance "/1 -> Sum3/2
  Integrator/1 -> Gain3/1, Gain1/1, Gain2/1  "X"
  Gain2/1 -> Demux/1
  Sum1/1 -> Sum3/1
  Step/1 -> Sum1/1
  Demux/1 -> Scope/1  "x"
  Demux/2 -> Scope/2  "error_y"

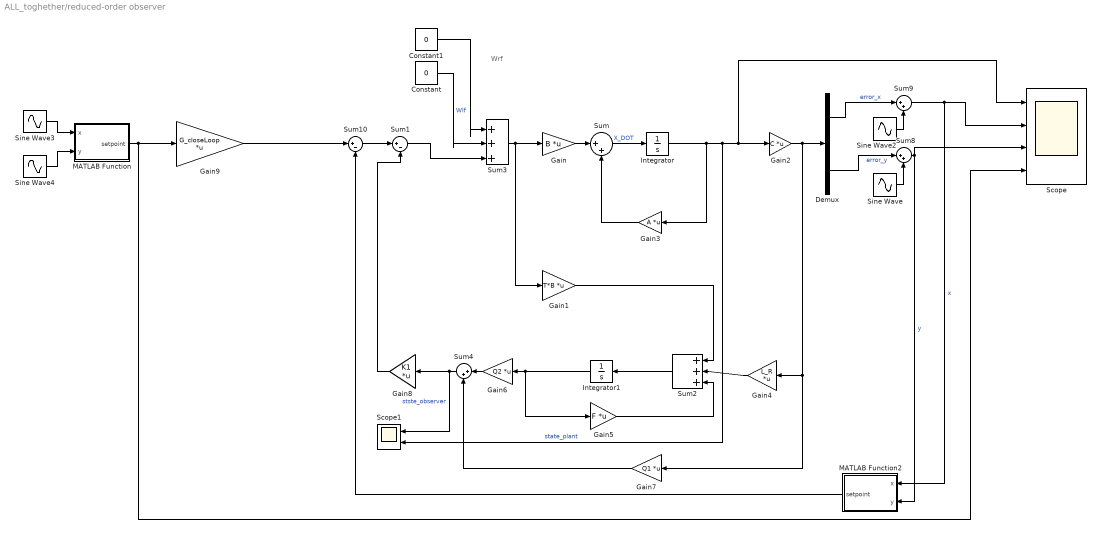
== system ALL_toghether/reduced-order observer ==
  note: Wrf
  Constant : Constant  Value=0
  Constant1 : Constant  Value=0
  Demux : Demux  Outputs=2
  Gain : Gain  Gain=B  Multiplication=Matrix(K*u)
  Gain1 : Gain  Gain=T*B  Multiplication=Matrix(K*u)
  Gain2 : Gain  Gain=C  Multiplication=Matrix(K*u)
  Gain3 : Gain  Gain=A  Multiplication=Matrix(K*u)
  Gain4 : Gain  Gain=L_R  Multiplication=Matrix(K*u)
  Gain5 : Gain  Gain=F  Multiplication=Matrix(K*u)
  Gain6 : Gain  Gain=Q2  Multiplication=Matrix(K*u)
  Gain7 : Gain  Gain=Q1  Multiplication=Matrix(K*u)
  Gain8 : Gain  Gain=K1  Multiplication=Matrix(K*u)
  Gain9 : Gain  Gain=G_closeLoop  Multiplication=Matrix(K*u)
  Integrator : Integrator  InitialCondition=[0.1 0.1 0]'
  Integrator1 : Integrator  InitialCondition=0.05
  MATLAB Function : MATLAB Function  TreatAsAtomicUnit=on
  MATLAB Function2 : MATLAB Function  TreatAsAtomicUnit=on
  Scope : Scope  NumInputPorts=4
  Scope1 : Scope  NumInputPorts=2
  Sine Wave : Sin  Amplitude=-3  Frequency=pi/16  SampleTime=0
  Sine Wave2 : Sin  Amplitude=3  Frequency=pi/16  Phase=pi/2  SampleTime=0
  Sine Wave3 : Sin  Amplitude=3  Frequency=pi/16  Phase=pi/2  SampleTime=0
  Sine Wave4 : Sin  Amplitude=-3  Frequency=pi/16  SampleTime=0
  Sum{,4,8..9} (4 alike) : Sum  Inputs=|++
  Sum1 : Sum  Inputs=|+-
  Sum10 : Sum  Inputs=|+-
  Sum2 : Sum  Inputs=|+++
  Sum3 : Sum  Inputs=|+++
  wires:
  Sum10/1 -> Sum1/1
  Constant/1 -> Sum3/2  "Wlf"
  Sum8/1 -> MATLAB Function2/2(y), Scope/3  "y"
  Sine Wave3/1 -> MATLAB Function/1(x)
  Sine Wave/1 -> Sum8/2
  Sum/1 -> Integrator/1  "X_DOT"
  Sine Wave4/1 -> MATLAB Function/2(y)
  Integrator/1 -> Gain3/1, Scope1/2, Scope/1, Gain2/1  "state_plant"
  Gain2/1 -> Gain7/1, Gain4/1, Demux/1
  Demux/2 -> Sum8/1  "error_y"
  Demux/1 -> Sum9/1  "error_x"
  Gain3/1 -> Sum/2
  MATLAB Function2/1(setpoint) -> Sum10/2
  Gain/1 -> Sum/1
  Sum9/1 -> MATLAB Function2/1(x), Scope/2  "x"
  Sum1/1 -> Sum3/3
  Sum3/1 -> Gain1/1, Gain/1
  Sine Wave2/1 -> Sum9/2
  Constant1/1 -> Sum3/1
  Sum2/1 -> Integrator1/1
  Gain5/1 -> Sum2/3
  Integrator1/1 -> Gain5/1, Gain6/1
  Gain4/1 -> Sum2/2
  Gain1/1 -> Sum2/1
  Gain6/1 -> Sum4/1
  Gain7/1 -> Sum4/2
  Sum4/1 -> Scope1/1, Gain8/1  "stste_observer"
  Gain8/1 -> Sum1/2
  MATLAB Function/1(setpoint) -> Scope/4, Gain9/1
  Gain9/1 -> Sum10/1

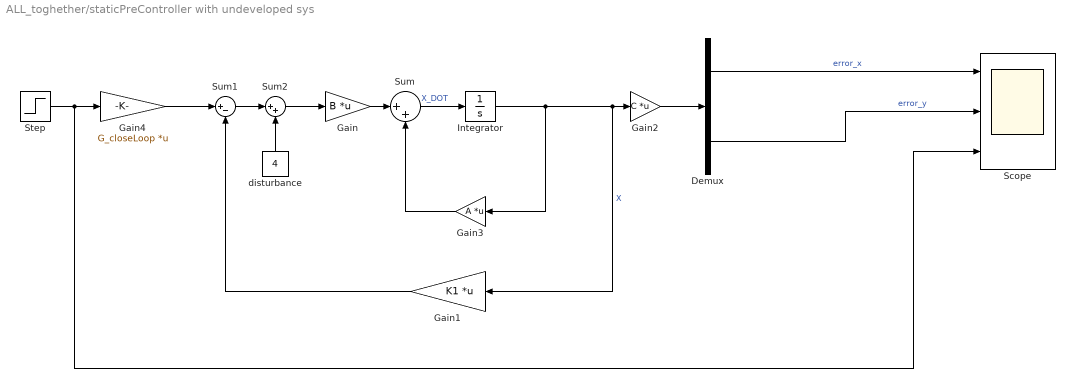
== system ALL_toghether/staticPreController with undeveloped sys ==
  Demux : Demux  Outputs=2
  Gain : Gain  Gain=B  Multiplication=Matrix(K*u)
  Gain1 : Gain  Gain=K1  Multiplication=Matrix(K*u)
  Gain2 : Gain  Gain=C  Multiplication=Matrix(K*u)
  Gain3 : Gain  Gain=A  Multiplication=Matrix(K*u)
  Gain4 : Gain  Gain=G_closeLoop  Multiplication=Matrix(K*u)
  Integrator : Integrator
  Scope : Scope  NumInputPorts=3
  Step : Step  Time=[0 0]'  Before=[0 0]'  After=[0.8 0.4]'  SampleTime=0
  Sum : Sum  Inputs=|++
  Sum1 : Sum  Inputs=|+-
  Sum2 : Sum  Inputs=|++
  "disturbance " : Constant  Value=4
  wires:
  Gain2/1 -> Demux/1
  Gain1/1 -> Sum1/2
  Integrator/1 -> Gain2/1, Gain1/1, Gain3/1  "X"
  Gain/1 -> Sum/1
  Sum/1 -> Integrator/1  "X_DOT"
  Gain3/1 -> Sum/2
  "disturbance "/1 -> Sum2/2
  Sum1/1 -> Sum2/1
  Sum2/1 -> Gain/1
  Demux/1 -> Scope/1  "error_x"
  Demux/2 -> Scope/2  "error_y"
  Gain4/1 -> Sum1/1
  Step/1 -> Scope/3, Gain4/1

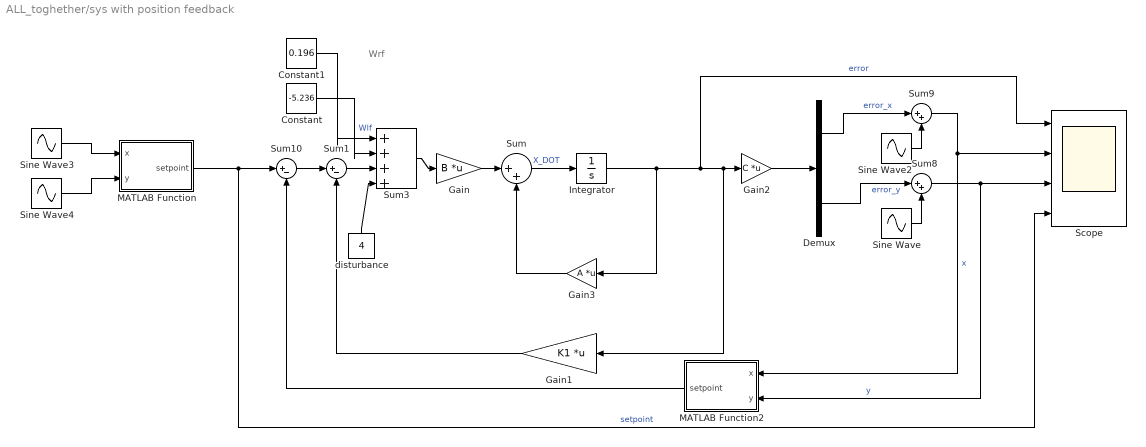
== system ALL_toghether/sys with position feedback ==
  note: Wrf
  Constant : Constant  Value=-5.236
  Constant1 : Constant  Value=0.196
  Demux : Demux  Outputs=2
  Gain : Gain  Gain=B  Multiplication=Matrix(K*u)
  Gain1 : Gain  Gain=K1  Multiplication=Matrix(K*u)
  Gain2 : Gain  Gain=C  Multiplication=Matrix(K*u)
  Gain3 : Gain  Gain=A  Multiplication=Matrix(K*u)
  Integrator : Integrator  InitialCondition=[0.1; 0.1; 0.1]
  MATLAB Function : MATLAB Function  TreatAsAtomicUnit=on
  MATLAB Function2 : MATLAB Function  TreatAsAtomicUnit=on
  Scope : Scope  NumInputPorts=4
  Sine Wave : Sin  Amplitude=-3  Frequency=pi/16  SampleTime=0
  Sine Wave2 : Sin  Amplitude=3  Frequency=pi/16  Phase=pi/2  SampleTime=0
  Sine Wave3 : Sin  Amplitude=3  Frequency=pi/16  Phase=pi/2  SampleTime=0
  Sine Wave4 : Sin  Amplitude=-3  Frequency=pi/16  SampleTime=0
  Sum : Sum  Inputs=|++
  Sum1 : Sum  Inputs=|+-
  Sum10 : Sum  Inputs=|+-
  Sum3 : Sum  Inputs=|++++
  Sum8 : Sum  Inputs=|++
  Sum9 : Sum  Inputs=|++
  "disturbance " : Constant  Value=4
  wires:
  Demux/2 -> Sum8/1  "error_y"
  MATLAB Function2/1(setpoint) -> Sum10/2
  Constant1/1 -> Sum3/1
  Sine Wave2/1 -> Sum9/2
  Sine Wave3/1 -> MATLAB Function/1(x)
  Sine Wave4/1 -> MATLAB Function/2(y)
  Constant/1 -> Sum3/2  "Wlf"
  Sum1/1 -> Sum3/3
  Sum/1 -> Integrator/1  "X_DOT"
  Sine Wave/1 -> Sum8/2
  Sum3/1 -> Gain/1
  "disturbance "/1 -> Sum3/4
  Gain1/1 -> Sum1/2
  Gain/1 -> Sum/1
  Integrator/1 -> Gain2/1, Gain1/1, Scope/1, Gain3/1  "error"
  MATLAB Function/1(setpoint) -> Sum10/1, Scope/4  "setpoint"
  Sum10/1 -> Sum1/1
  Gain2/1 -> Demux/1
  Sum8/1 -> Scope/3, MATLAB Function2/2(y)  "y"
  Gain3/1 -> Sum/2
  Sum9/1 -> Scope/2, MATLAB Function2/1(x)  "x"
  Demux/1 -> Sum9/1  "error_x"

== matlab function ALL_toghether/MAHYA /MATLAB Function2 ==
  data: x input; setpoint output; y input
function setpoint = fcn(x, y)

setpoint = [x; y];

== matlab function ALL_toghether/MAHYA /MATLAB Function1 ==
  data: u input; xh output; y input; z input; zd output
function [xh,zd] = fcn(u,y,z)
L_R = [1 5];
A=[0 -pi/16 0;pi/16 0 3*pi/16;0 0 0];
B=[1/2 1/2;0 0;1/0.15 -1/0.15];
C=[1 0 0;0 1 0];
F=[-40];
T=[];
T = lyap(F, A, -L_R*C);
zd = -40*z+T*B*u+L_R*y
xh=[1 0;0 1;0.0244 0.1251]*y+[0;0;-0.0018]*z

== matlab function ALL_toghether/MAHYA /MATLAB Function3 ==
  data: x input; setpoint output; y input
function setpoint = fcn(x, y)

setpoint = [x; y];

== matlab function ALL_toghether/sys with position feedback/MATLAB Function ==
  data: x input; setpoint output; y input
function setpoint = fcn(x, y)

setpoint = [x; y];

== matlab function ALL_toghether/phase4_sys with positionFeedback /MATLAB Function5 ==
  data: x input; setpoint output; y input
function setpoint = fcn(x, y)

setpoint = [x; y];

== matlab function ALL_toghether/sys with position feedback/MATLAB Function2 ==
  data: x input; setpoint output; y input
function setpoint = fcn(x, y)

setpoint = [x; y];

== matlab function ALL_toghether/phase4_fullOrderObserver /MATLAB Function ==
  data: x input; setpoint output; y input
function setpoint = fcn(x, y)

setpoint = [x; y];

== matlab function ALL_toghether/phase4_fullOrderObserver /MATLAB Function2 ==
  data: x input; setpoint output; y input
function setpoint = fcn(x, y)

setpoint = [x; y];

== matlab function ALL_toghether/phase4_fullOrderObserver /MATLAB Function1 ==
  data: x input; setpoint output; y input
function setpoint = fcn(x, y)

setpoint = [x; y];

== matlab function ALL_toghether/phase4_fullOrderObserver /MATLAB Function3 ==
  data: x input; setpoint output; y input
function setpoint = fcn(x, y)

setpoint = [x; y];

== matlab function ALL_toghether/MAHYA /MATLAB Function ==
  data: x input; setpoint output; y input
function setpoint = fcn(x, y)

setpoint = [x; y];

== matlab function ALL_toghether/phase4_fullOrderObserver /MATLAB Function4 ==
  data: x input; setpoint output; y input
function setpoint = fcn(x, y)

setpoint = [x; y];

== matlab function ALL_toghether/phase4_fullOrderObserver /MATLAB Function5 ==
  data: x input; setpoint output; y input
function setpoint = fcn(x, y)

setpoint = [x; y];

== matlab function ALL_toghether/phase4_reducedOrderObserver /MATLAB Function ==
  data: x input; setpoint output; y input
function setpoint = fcn(x, y)

setpoint = [x; y];

== matlab function ALL_toghether/phase4_reducedOrderObserver /MATLAB Function2 ==
  data: x input; setpoint output; y input
function setpoint = fcn(x, y)

setpoint = [x; y];

== matlab function ALL_toghether/phase4_reducedOrderObserver /MATLAB Function1 ==
  data: x input; setpoint output; y input
function setpoint = fcn(x, y)

setpoint = [x; y];

== matlab function ALL_toghether/phase4_reducedOrderObserver /MATLAB Function3 ==
  data: x input; setpoint output; y input
function setpoint = fcn(x, y)

setpoint = [x; y];

== matlab function ALL_toghether/phase4_reducedOrderObserver /MATLAB Function4 ==
  data: x input; setpoint output; y input
function setpoint = fcn(x, y)

setpoint = [x; y];

== matlab function ALL_toghether/phase4_reducedOrderObserver /MATLAB Function5 ==
  data: x input; setpoint output; y input
function setpoint = fcn(x, y)

setpoint = [x; y];

== matlab function ALL_toghether/phase4_sys with positionFeedback /MATLAB Function ==
  data: x input; setpoint output; y input
function setpoint = fcn(x, y)

setpoint = [x; y];

== matlab function ALL_toghether/phase4_sys with positionFeedback /MATLAB Function2 ==
  data: x input; setpoint output; y input
function setpoint = fcn(x, y)

setpoint = [x; y];

== matlab function ALL_toghether/nonlinear sys /MATLAB Function1 ==
  data: e input; U input; e_dot output
function e_dot  = fcn(e,U)
e_dot = [0.1;-0.1;0.05]; 
theta_dot_ref = -(pi/16) ;
v_ref = 3*(pi/16) ;
e_dot(1)=(theta_dot_ref - U(1))*e(2) + v_ref*cos(e(3))+(U(2) - v_ref);
e_dot(2)=(U(1)-theta_dot_ref)*e(1) + v_ref*sin(e(3));
e_dot(3)= U(1);

== matlab function ALL_toghether/phase4_sys with positionFeedback /MATLAB Function1 ==
  data: x input; setpoint output; y input
function setpoint = fcn(x, y)

setpoint = [x; y];

== matlab function ALL_toghether/full-order observer /MATLAB Function ==
  data: x input; setpoint output; y input
function setpoint = fcn(x, y)

setpoint = [x; y];

== matlab function ALL_toghether/full-order observer /MATLAB Function2 ==
  data: x input; setpoint output; y input
function setpoint = fcn(x, y)

setpoint = [x; y];

== matlab function ALL_toghether/reduced-order observer/MATLAB Function ==
  data: x input; setpoint output; y input
function setpoint = fcn(x, y)

setpoint = [x; y];

== matlab function ALL_toghether/reduced-order observer/MATLAB Function2 ==
  data: x input; setpoint output; y input
function setpoint = fcn(x, y)

setpoint = [x; y];

== matlab function ALL_toghether/phase4_sys with positionFeedback /MATLAB Function3 ==
  data: x input; setpoint output; y input
function setpoint = fcn(x, y)

setpoint = [x; y];

== matlab function ALL_toghether/phase4_sys with positionFeedback /MATLAB Function4 ==
  data: x input; setpoint output; y input
function setpoint = fcn(x, y)

setpoint = [x; y];
